simulink model "DRU24_PowerFactor"  (Simulink 7.9)
settings: Solver=ode45  StartTime=0.0  StopTime=1  RelTol=1e-3
undefined symbols (not defined in the file or in its folder): D1, Delta
libraries: powerlib x38
settings Model: Creator=H002220  LastModifiedBy=H002220

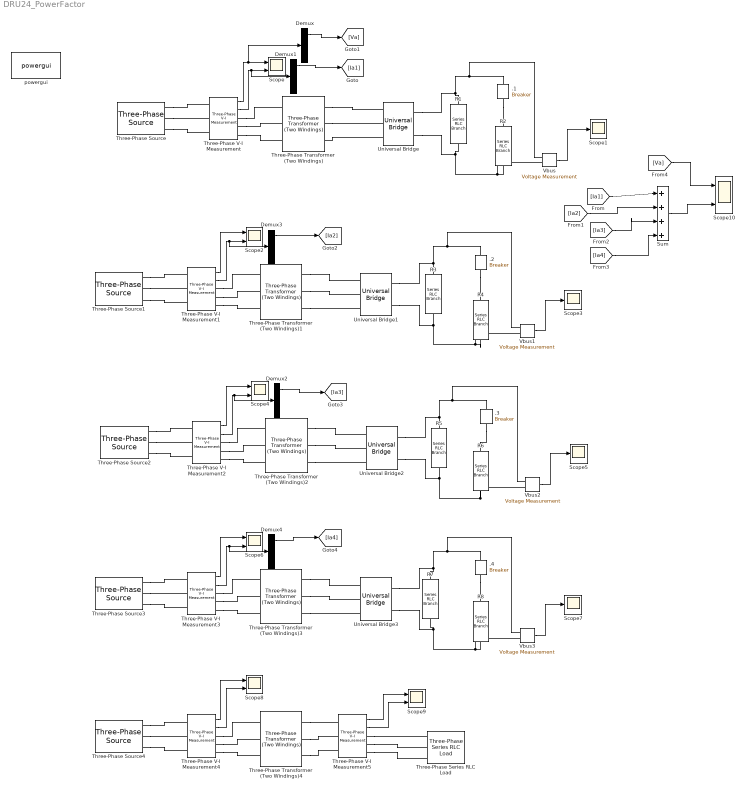
== system DRU24_PowerFactor ==
  .{1..4} (4 alike) : powerlib/Elements/Breaker  BreakerResistance=0.001  InitialState=0  SnubberResistance=1e6  SnubberCapacitance=inf  SwitchingTimes=[0.5]  External=off  Measurements=None  MoreParameters=off  NoBreakLoop=off
      settings: AttributesFormatString=\n
  Demux{,1..4} (5 alike) : Demux  Outputs=3
  R{1,3,5,7} (4 alike) : powerlib/Elements/Series RLC Branch  LConnTagsString=__new0  RConnTagsString=__new0  BranchType=C  Resistance=1e4  Inductance=1e-3  SetiL0=off  InitialCurrent=0  Capacitance=2000e-6  Setx0=off  InitialVoltage=0  Measurements=None
  R{2,4,6,8} (4 alike) : powerlib/Elements/Series RLC Branch  LConnTagsString=__new0  RConnTagsString=__new0  BranchType=R  Resistance=87.55  Inductance=1e-3  SetiL0=off  InitialCurrent=0  Capacitance=1e-6  Setx0=off  InitialVoltage=0  Measurements=None
  Scope{,2,4,6,8..10} (7 alike) : Scope  NumInputPorts=2
      Scope settings: YMin=-5~-5  YMax=5~5
      Scope10 settings: YMin=-40000~-260  YMax=40000~260  SaveName=ScopeData10
      Scope2 settings: YMin=-5~-5  YMax=5~5  SaveName=ScopeData2
      Scope4 settings: YMin=-5~-5  YMax=5~5  SaveName=ScopeData4
      Scope6 settings: YMin=-5~-5  YMax=5~5  SaveName=ScopeData6
      Scope8 settings: YMin=-5~-5  YMax=5~5  SaveName=ScopeData8
      Scope9 settings: YMin=-5~-5  YMax=5~5  SaveName=ScopeData9
  Scope{1,3,5,7} (4 alike) : Scope
      Scope3 settings: SaveName=ScopeData3
      Scope5 settings: SaveName=ScopeData5
      Scope7 settings: SaveName=ScopeData7
  Sum : Sum  Inputs=|++++
  Three-Phase Series RLC Load : powerlib/Elements/Three-Phase Series RLC Load  LConnTagsString=A|B|C  Configuration=Y (grounded)  NominalVoltage=1800  NominalFrequency=50  ActivePower=1e6  InductivePower=0  CapacitivePower=0  Measurements=None  LoadType=constant Z
  Three-Phase Transformer (Two Windings) : powerlib/Elements/Three-Phase Transformer (Two Windings)  Winding1Connection=Delta (D1)  UNITS=pu  NominalPower=[ 1.25e6 , 50 ]  Winding1=[ 25e3 , 0.002 , 0.01 ]  Winding2Connection=Delta (D1)  Winding2=[ 1.8e3 , 0.002 , 0.064 ]  SetSaturation=off  Rm=500  Lm=500  Saturation=[ 0,0 ; 0.0024,1.2 ; 1.0,1.52 ]  Hysteresis=off  DataFile='hysteresis'  SetInitialFlux=off  InitialFluxes=[ 0.8 , -0.8 , 0.7 ]  Measurements=None  MoreParameters=off  BreakLoop=off  DataType=off  TransfoNumber=1
  Three-Phase Transformer (Two Windings)1 : powerlib/Elements/Three-Phase Transformer (Two Windings)  Winding1Connection=Delta (D1)  UNITS=pu  NominalPower=[ 1.25e6 , 50 ]  Winding1=[ 25e3 , 0.002 , 0.01 ]  Winding2Connection=Delta (D1)  Winding2=[ 1.8e3 , 0.002 , 0.064 ]  SetSaturation=off  Rm=500  Lm=500  Saturation=[ 0,0 ; 0.0024,1.2 ; 1.0,1.52 ]  Hysteresis=off  DataFile='hysteresis'  SetInitialFlux=off  InitialFluxes=[ 0.8 , -0.8 , 0.7 ]  Measurements=None  MoreParameters=off  BreakLoop=off  DataType=off  TransfoNumber=1
  Three-Phase Transformer (Two Windings)2 : powerlib/Elements/Three-Phase Transformer (Two Windings)  Winding1Connection=Delta (D1)  UNITS=pu  NominalPower=[ 1.25e6 , 50 ]  Winding1=[ 25e3 , 0.002 , 0.01 ]  Winding2Connection=Delta (D1)  Winding2=[ 1.8e3 , 0.002 , 0.064 ]  SetSaturation=off  Rm=500  Lm=500  Saturation=[ 0,0 ; 0.0024,1.2 ; 1.0,1.52 ]  Hysteresis=off  DataFile='hysteresis'  SetInitialFlux=off  InitialFluxes=[ 0.8 , -0.8 , 0.7 ]  Measurements=None  MoreParameters=off  BreakLoop=off  DataType=off  TransfoNumber=1
  Three-Phase Transformer (Two Windings)3 : powerlib/Elements/Three-Phase Transformer (Two Windings)  Winding1Connection=Delta (D1)  UNITS=pu  NominalPower=[ 1.25e6 , 50 ]  Winding1=[ 25e3 , 0.002 , 0.01 ]  Winding2Connection=Delta (D1)  Winding2=[ 1.8e3 , 0.002 , 0.15 ]  SetSaturation=off  Rm=500  Lm=500  Saturation=[ 0,0 ; 0.0024,1.2 ; 1.0,1.52 ]  Hysteresis=off  DataFile='hysteresis'  SetInitialFlux=off  InitialFluxes=[ 0.8 , -0.8 , 0.7 ]  Measurements=None  MoreParameters=off  BreakLoop=off  DataType=off  TransfoNumber=1
  Three-Phase Transformer (Two Windings)4 : powerlib/Elements/Three-Phase Transformer (Two Windings)  Winding1Connection=Delta (D1)  UNITS=pu  NominalPower=[ 1.25e6 , 50 ]  Winding1=[ 25e3 , 0.002 , 0.01 ]  Winding2Connection=Y  Winding2=[ 1.8e3 , 0.002 , 0.064 ]  SetSaturation=off  Rm=500  Lm=500  Saturation=[ 0,0 ; 0.0024,1.2 ; 1.0,1.52 ]  Hysteresis=off  DataFile='hysteresis'  SetInitialFlux=off  InitialFluxes=[ 0.8 , -0.8 , 0.7 ]  Measurements=None  MoreParameters=off  BreakLoop=off  DataType=off  TransfoNumber=1
  Three-Phase V-I Measurement{,1..3} (4 alike) : powerlib/Measurements/Three-Phase V-I Measurement  VoltageMeasurement=phase-to-phase  SetLabelV=off  LabelV=Vabc  Vpu=off  VpuLL=off  CurrentMeasurement=yes  SetLabelI=off  LabelI=Iabc  Ipu=off  Pbase=100e6  Vbase=500e3  OutputType=Complex  PhasorSimulation=off  PSBequivalent=0
  Three-Phase V-I Measurement4 : powerlib/Measurements/Three-Phase V-I Measurement  VoltageMeasurement=phase-to-ground  SetLabelV=off  LabelV=Vabc  Vpu=off  VpuLL=off  CurrentMeasurement=yes  SetLabelI=off  LabelI=Iabc  Ipu=off  Pbase=100e6  Vbase=500e3  OutputType=Complex  PhasorSimulation=off  PSBequivalent=0
  Three-Phase V-I Measurement5 : powerlib/Measurements/Three-Phase V-I Measurement  VoltageMeasurement=phase-to-ground  SetLabelV=off  LabelV=Vabc  Vpu=off  VpuLL=off  CurrentMeasurement=yes  SetLabelI=off  LabelI=Iabc  Ipu=off  Pbase=100e6  Vbase=500e3  OutputType=Complex  PhasorSimulation=off  PSBequivalent=0
  Three-Phase Source : powerlib/Electrical Sources/Three-Phase Source  Voltage=25e3  PhaseAngle=0  Frequency=50  InternalConnection=Yg  SpecifyImpedance=off  Resistance=1e-5  Inductance=1e-6  ShortCircuitLevel=1e8  BaseVoltage=25e3  XRratio=0.1  BusType=swing  Pref=0  Qref=0  Qmin=-inf  Qmax=inf
  Three-Phase Source1 : powerlib/Electrical Sources/Three-Phase Source  Voltage=25e3  PhaseAngle=15  Frequency=50  InternalConnection=Yg  SpecifyImpedance=off  Resistance=1e-5  Inductance=1e-6  ShortCircuitLevel=1e8  BaseVoltage=25e3  XRratio=0.1  BusType=swing  Pref=0  Qref=0  Qmin=-inf  Qmax=inf
  Three-Phase Source2 : powerlib/Electrical Sources/Three-Phase Source  Voltage=25e3  PhaseAngle=30  Frequency=50  InternalConnection=Yg  SpecifyImpedance=off  Resistance=1e-5  Inductance=1e-6  ShortCircuitLevel=1e8  BaseVoltage=25e3  XRratio=0.1  BusType=swing  Pref=0  Qref=0  Qmin=-inf  Qmax=inf
  Three-Phase Source3 : powerlib/Electrical Sources/Three-Phase Source  Voltage=25e3  PhaseAngle=45  Frequency=50  InternalConnection=Yg  SpecifyImpedance=off  Resistance=1e-5  Inductance=1e-6  ShortCircuitLevel=1e8  BaseVoltage=25e3  XRratio=0.1  BusType=swing  Pref=0  Qref=0  Qmin=-inf  Qmax=inf
  Three-Phase Source4 : powerlib/Electrical Sources/Three-Phase Source  Voltage=25e3  PhaseAngle=0  Frequency=50  InternalConnection=Yg  SpecifyImpedance=off  Resistance=1e-5  Inductance=1e-6  ShortCircuitLevel=1e8  BaseVoltage=25e3  XRratio=0.1  BusType=swing  Pref=0  Qref=0  Qmin=-inf  Qmax=inf
  Universal Bridge{,1..3} (4 alike) : powerlib/Power Electronics/Universal Bridge  Arms=3  SnubberResistance=1e5  SnubberCapacitance=inf  Device=Diodes  Ron=1e-3  Lon=0  ForwardVoltages="[  0  0  ]"  ForwardVoltage=0.2  GTOparameters=[ 10e-6 , 20e-6 ]  IGBTparameters=[ 1e-6 , 2e-6 ]  Measurements=None  Measurements_2=None  converterType=Rectifier
  Vbus{,1..3} (4 alike) : powerlib/Measurements/Voltage Measurement  PhasorSimulation=off  OutputType=Complex  PSBequivalent=0
  powergui : powerlib/powergui  Priority=2  SimulationMode=Discrete  SolverType=Tustin  SampleTime=50e-6  frequency=60  SPID=off  DisableSnubberDevices=off  DisableRonSwitches=off  DisableVfSwitches=off  SwTol=0  Interpol=off  DisplayEquations=off  FunctionMessages=off  frequencyindice=50  Pbase=100e6  ErrMax=1e-4  Iterations=50  UnitsV=kV  UnitsW=MW  echomessages=off  HookPort=off  EnableUseOfTLC=off  x0status=blocks  RestoreLinks=warning  ResistiveCurrentMeasurement=off  Frange=[0:2:500]  Ylog=off  Xlog=on  ShowGrid=off  save=off  variable=ZData  structure=ScopeData10  ZoomFFT=off  StartTime=0.98  cycles=1  DisplayStyle=2  fundamental=50  FreqAxis=on  MaxFrequency=1000  frequencyindicesteady=1  RmsSteady=1  display=off  Ts=0  methode=off
  wires:
  Three-Phase V-I Measurement/2 -> Scope/2, Demux1/1
  Three-Phase V-I Measurement/1 -> Scope/1, Demux/1
  Vbus/1 -> Scope1/1
  Demux1/1 -> [Ia1]
  Demux/1 -> [Va]
  Three-Phase V-I Measurement1/2 -> Demux3/1, Scope2/2
  Three-Phase V-I Measurement1/1 -> Scope2/1
  Vbus1/1 -> Scope3/1
  Demux3/1 -> [Ia2]
  Three-Phase V-I Measurement2/2 -> Scope4/2, Demux2/1
  Three-Phase V-I Measurement2/1 -> Scope4/1
  Vbus2/1 -> Scope5/1
  Demux2/1 -> [Ia3]
  Three-Phase V-I Measurement3/2 -> Demux4/1, Scope6/2
  Three-Phase V-I Measurement3/1 -> Scope6/1
  Vbus3/1 -> Scope7/1
  Demux4/1 -> [Ia4]
  Three-Phase V-I Measurement4/2 -> Scope8/2
  Three-Phase V-I Measurement4/1 -> Scope8/1
  Three-Phase V-I Measurement5/2 -> Scope9/2
  Three-Phase V-I Measurement5/1 -> Scope9/1
  [Ia1] -> Sum/1
  [Ia2] -> Sum/2
  [Ia3] -> Sum/3
  [Ia4] -> Sum/4
  Sum/1 -> Scope10/2
  [Va] -> Scope10/1
  connections:
  Three-Phase Source/RConn1 -- Three-Phase V-I Measurement/LConn1
  Three-Phase Source/RConn2 -- Three-Phase V-I Measurement/LConn2
  Three-Phase Source/RConn3 -- Three-Phase V-I Measurement/LConn3
  Three-Phase V-I Measurement/RConn2 -- Three-Phase Transformer (Two Windings)/LConn2
  Three-Phase V-I Measurement/RConn1 -- Three-Phase Transformer (Two Windings)/LConn1
  Three-Phase V-I Measurement/RConn3 -- Three-Phase Transformer (Two Windings)/LConn3
  Three-Phase Transformer (Two Windings)/RConn1 -- Universal Bridge/LConn1
  Three-Phase Transformer (Two Windings)/RConn2 -- Universal Bridge/LConn2
  Three-Phase Transformer (Two Windings)/RConn3 -- Universal Bridge/LConn3
  Universal Bridge/RConn1 -- R1/LConn1 -- .1/LConn1 -- Vbus/LConn1
  R2/RConn1 -- Vbus/LConn2 -- Universal Bridge/RConn2 -- R1/RConn1
  .1/RConn1 -- R2/LConn1
  R4/RConn1 -- Vbus1/LConn2 -- R3/RConn1 -- Universal Bridge1/RConn2
  Three-Phase Source1/RConn1 -- Three-Phase V-I Measurement1/LConn1
  Three-Phase Source1/RConn2 -- Three-Phase V-I Measurement1/LConn2
  Three-Phase Source1/RConn3 -- Three-Phase V-I Measurement1/LConn3
  Three-Phase V-I Measurement1/RConn2 -- Three-Phase Transformer (Two Windings)1/LConn2
  Three-Phase V-I Measurement1/RConn1 -- Three-Phase Transformer (Two Windings)1/LConn1
  Three-Phase V-I Measurement1/RConn3 -- Three-Phase Transformer (Two Windings)1/LConn3
  .2/RConn1 -- R4/LConn1
  Three-Phase Transformer (Two Windings)1/RConn3 -- Universal Bridge1/LConn3
  Three-Phase Transformer (Two Windings)1/RConn2 -- Universal Bridge1/LConn2
  Three-Phase Transformer (Two Windings)1/RConn1 -- Universal Bridge1/LConn1
  R5/LConn1 -- .3/LConn1 -- Vbus2/LConn1 -- Universal Bridge2/RConn1
  R5/RConn1 -- R6/RConn1 -- Vbus2/LConn2 -- Universal Bridge2/RConn2
  Three-Phase Source2/RConn3 -- Three-Phase V-I Measurement2/LConn3
  Three-Phase Transformer (Two Windings)2/RConn2 -- Universal Bridge2/LConn2
  Three-Phase V-I Measurement2/RConn2 -- Three-Phase Transformer (Two Windings)2/LConn2
  Three-Phase Transformer (Two Windings)2/RConn3 -- Universal Bridge2/LConn3
  .3/RConn1 -- R6/LConn1
  Three-Phase V-I Measurement2/RConn1 -- Three-Phase Transformer (Two Windings)2/LConn1
  Three-Phase Transformer (Two Windings)2/RConn1 -- Universal Bridge2/LConn1
  Three-Phase Source2/RConn1 -- Three-Phase V-I Measurement2/LConn1
  Three-Phase Source2/RConn2 -- Three-Phase V-I Measurement2/LConn2
  Three-Phase V-I Measurement2/RConn3 -- Three-Phase Transformer (Two Windings)2/LConn3
  .4/LConn1 -- R7/LConn1 -- Universal Bridge3/RConn1 -- Vbus3/LConn1
  R8/RConn1 -- R7/RConn1 -- Universal Bridge3/RConn2 -- Vbus3/LConn2
  Three-Phase V-I Measurement3/RConn3 -- Three-Phase Transformer (Two Windings)3/LConn3
  Three-Phase Source3/RConn1 -- Three-Phase V-I Measurement3/LConn1
  Three-Phase Transformer (Two Windings)3/RConn3 -- Universal Bridge3/LConn3
  Three-Phase V-I Measurement3/RConn2 -- Three-Phase Transformer (Two Windings)3/LConn2
  Three-Phase Source3/RConn3 -- Three-Phase V-I Measurement3/LConn3
  Three-Phase Transformer (Two Windings)3/RConn2 -- Universal Bridge3/LConn2
  Three-Phase V-I Measurement3/RConn1 -- Three-Phase Transformer (Two Windings)3/LConn1
  Three-Phase Source3/RConn2 -- Three-Phase V-I Measurement3/LConn2
  Three-Phase Transformer (Two Windings)3/RConn1 -- Universal Bridge3/LConn1
  .4/RConn1 -- R8/LConn1
  Three-Phase V-I Measurement4/RConn1 -- Three-Phase Transformer (Two Windings)4/LConn1
  Three-Phase V-I Measurement4/RConn3 -- Three-Phase Transformer (Two Windings)4/LConn3
  Three-Phase Source4/RConn3 -- Three-Phase V-I Measurement4/LConn3
  Three-Phase V-I Measurement4/RConn2 -- Three-Phase Transformer (Two Windings)4/LConn2
  Three-Phase Source4/RConn2 -- Three-Phase V-I Measurement4/LConn2
  Three-Phase Source4/RConn1 -- Three-Phase V-I Measurement4/LConn1
  Three-Phase Transformer (Two Windings)4/RConn1 -- Three-Phase V-I Measurement5/LConn1
  Three-Phase Transformer (Two Windings)4/RConn2 -- Three-Phase V-I Measurement5/LConn2
  Three-Phase Transformer (Two Windings)4/RConn3 -- Three-Phase V-I Measurement5/LConn3
  Three-Phase V-I Measurement5/RConn1 -- Three-Phase Series RLC Load/LConn1
  Three-Phase V-I Measurement5/RConn2 -- Three-Phase Series RLC Load/LConn2
  Three-Phase V-I Measurement5/RConn3 -- Three-Phase Series RLC Load/LConn3
  Universal Bridge1/RConn1 -- R3/LConn1 -- Vbus1/LConn1 -- .2/LConn1
